simulink model "buenoensam"  (R2013a)
settings: Solver=ode5  StartTime=0.0  StopTime=40  FixedStep=.01  RelTol=1e-3
values from neighbouring files (symbols this model uses):
  g = 9.81    [miosinlazoalgebraico1.m]    (also in proyectoy6.m)
  theta2 = (m2*lc2*lc2)+I2    (= 0.00775807)    [miosinlazoalgebraico1.m]    (also in proyectoy6.m = 0.00125168)
  theta3 = (m2*l1*lc2)    (= 0.008897)    [miosinlazoalgebraico1.m]    (also in proyectoy6.m = 0.00091872)
  theta4 = (m1*lc1)+(m2*l1)    (= 0.495148)    [miosinlazoalgebraico1.m]    (also in proyectoy6.m = 0.014993)
  theta5 = (m2*lc2)    (= 0.044485)    [miosinlazoalgebraico1.m]    (also in proyectoy6.m = 0.008352)
undefined symbols (not defined in the file or in its folder): base, buenoensam, Pieza2, Pieza3, RootGround, RootPart, theta1
libraries: mblibv1 x14, fuzblock x4
settings Model: Creator=Daniel  LastModifiedBy=Daniel
settings SolverCC: MaxConsecutiveZCs=100000
settings SimMechanicsCC: VisOnUpdateDiagram=on  VisDuringSimulation=on

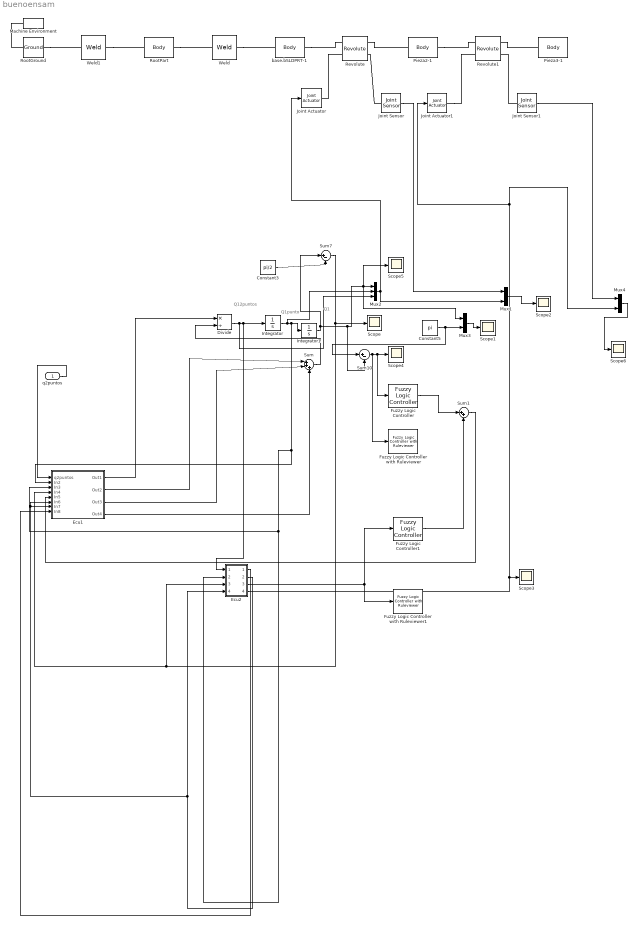
== system buenoensam ==
  note: Q1
  note: Q1punto
  note: Q12puntos
  q2puntos : Inport
  Constant3 : Constant  Value=pi/2
  Constant5 : Constant  Value=pi
  Divide : Product  Inputs=*/
  Ecu1 : Subsystem
  Ecu2 : Subsystem
  Fuzzy Logic Controller : fuzblock/Fuzzy Logic  Controller  fis=wero2P1
  Fuzzy Logic Controller with Ruleviewer : fuzblock/Fuzzy Logic  Controller  with Ruleviewer  fismatrix=wero2P1  Ts=2
  Fuzzy Logic Controller with Ruleviewer1 : fuzblock/Fuzzy Logic  Controller  with Ruleviewer  fismatrix=wero2P2  Ts=2
  Fuzzy Logic Controller1 : fuzblock/Fuzzy Logic  Controller  fis=wero2P2
  Integrator : Integrator
  Integrator1 : Integrator
  Joint Actuator : mblibv1/Sensors &  Actuators/Joint Actuator  UpdateFromCAD=off  PhysicalDomain=Mechanical  PortType=blob  ActuationStyle=Motion  AngleUnits=rad  ArcVelocityUnits=rad/s  ArcAccelerationUnits=rad/s^2  CoordPositionUnits=m  VelocityUnits=m/s  AccelerationUnits=m/s^2  ForceUnits=N  TorqueUnits=N*m  ActiveIO=on  Width=3  DialogClass=MechanicalActuatorBlock  Primitive=R1  ReferenceFrame=Absolute (World)
  Joint Actuator1 : mblibv1/Sensors &  Actuators/Joint Actuator  UpdateFromCAD=off  PhysicalDomain=Mechanical  PortType=blob  ActuationStyle=Motion  AngleUnits=rad  ArcVelocityUnits=rpm  ArcAccelerationUnits=rad/s^2  CoordPositionUnits=m  VelocityUnits=m/s  AccelerationUnits=m/s^2  ForceUnits=N  TorqueUnits=N*m  ActiveIO=on  Width=3  DialogClass=MechanicalActuatorBlock  Primitive=R1  ReferenceFrame=Absolute (World)
  Joint Sensor : mblibv1/Sensors &  Actuators/Joint Sensor  UpdateFromCAD=off  PhysicalDomain=Mechanical  PortType=blob  Muxed=on  Pose=off  Angle=on  AngleUnits=rad  ArcVelocity=off  ArcVelocityUnits=deg/s  ArcAcceleration=off  ArcAccelerationUnits=deg/s^2  CoordPosition=on  CoordPositionUnits=m  Velocity=off  VelocityUnits=m/s  Acceleration=off  AccelerationUnits=m/s^2  Quaternion=on  QuaternionDT=off  QuaternionDDT=off  QuaternionUnits=off  OutputVector=[1]  ActiveIO=on  Width=1  DialogClass=MechanicalSensorBlock  Primitive=R1  Force=off  ForceUnits=N  Torque=off  TorqueUnits=N*m  ReferenceFrame=Absolute (World)  ReactionSensedSide=Base  ReactionReferenceFrame=Absolute (World)  ReactionForce=off  ReactionForceUnits=N  ReactionMoment=off  ReactionMomentUnits=N*m
  Joint Sensor1 : mblibv1/Sensors &  Actuators/Joint Sensor  UpdateFromCAD=off  PhysicalDomain=Mechanical  PortType=blob  Muxed=on  Pose=off  Angle=on  AngleUnits=deg  ArcVelocity=off  ArcVelocityUnits=deg/s  ArcAcceleration=off  ArcAccelerationUnits=deg/s^2  CoordPosition=on  CoordPositionUnits=m  Velocity=off  VelocityUnits=m/s  Acceleration=off  AccelerationUnits=m/s^2  Quaternion=on  QuaternionDT=off  QuaternionDDT=off  QuaternionUnits=off  OutputVector=[1]  ActiveIO=on  Width=1  DialogClass=MechanicalSensorBlock  Primitive=R1  Force=off  ForceUnits=N  Torque=off  TorqueUnits=N-m  ReferenceFrame=Absolute (World)  ReactionSensedSide=Base  ReactionReferenceFrame=Absolute (World)  ReactionForce=off  ReactionForceUnits=N  ReactionMoment=off  ReactionMomentUnits=N-m
  Machine Environment : mblibv1/Bodies/Machine Environment  PortType=env  PhysicalDomain=Mechanical  DialogTemplateClass=MECH.MachineEnvironment  SyncWhenCopied=off  Gravity=[0 -9.81 0]  GravityUnits=m/s^2  GravityAsSignal=off  Dimensionality=Auto-detect  AnalysisType=Forward dynamics  LinearAssemblyTolerance=1e-3  LinearAssemblyToleranceUnits=m  AngularAssemblyTolerance=1e-3  AngularAssemblyToleranceUnits=rad  ConstraintSolverType=Stabilizing  ConstraintRelTolerance=1e-4  ConstraintAbsTolerance=1e-4  UseRobustSingularityHandling=off  RedundancyAnalysisToleranceType=Automatically select tolerance  RedundancyAnalysisTolerance=1e-14  StatePerturbationType=Fixed  PerturbationSize=1e-5  VisualizeMachine=on  BodyVisualizationType=Use model default body geometries  BodyColorSelMode=Use model default  DefaultBodyColor=[1 0 0]
  Mux1 : Mux  Inputs=2
  Mux2 : Mux  Inputs=3
  Mux3 : Mux  Inputs=2
  Mux4 : Mux  Inputs=2
  Pieza2-1 : mblibv1/Bodies/Body  LConnTagsString=CS2  RConnTagsString=CS3  UpdateFromCAD=on  PMImportedID=Pieza2-1  DialogClass=MechanicalBodyBlock  Mass=0.734204  MassUnits=kg  InertiaUnits=kg*m^2  Inertia=[0.000264247,2.83059e-10,-6.28102e-08;2.83059e-10,0.0127231,5.8833e-11;-6.28102e-08,5.8833e-11,0.0126365]  Shape=Cylinder  ShapeDims=[1 1]  ShapeUnits=m  ShapeUse=false  Density=1  DensityUnits=kg/m^3  DensityUse=false  GraphicsMode=GFXFILE  GraphicsFileName=buenoensam - Pieza2-1.STL  BodyColorSelMode=COLORPALETTE  BodyColor=[1;1;0]  AttachedToCS=CS1  CG=Right$CG$[-0.0307943 -0.183465 0.38735]$WORLD$WORLD$m$[0.0349053 0 -0.999391;-0.999391 0 -0.0349053;0 1 0]$3x3 Transform$rad$WORLD$false$Pieza2-1::CG(AUTOGEN)  WorkingFrames=Right$CS1$[-0.0615922 -0.0278733 0.3683]$WORLD$WORLD$m$[0.0349053 0 -0.999391;-0.999391 0 -0.0349053;0 1 0]$3x3 Transform$rad$WORLD$false$Pieza2-1::CS1(AUTOGEN)#Left$CS2$[-0.0384461 0.0361919 0.3683]$WORLD$WORLD$m$[1 0 0;0 1 0;0 0 1]$3x3 Transform$rad$WORLD$true$Pieza2-1:-:base.bSLDPRT-1::Pieza2-1(AUTOGEN)#Right$CS3$[-0.0234804 -0.394088 0.3683]$WORLD$WORLD$m$[1 0 0;0 1 0;0 0 1]$3x3 Transform$rad$WORLD$true$Pieza2-1:-:Pieza3-1::Pieza2-1(AUTOGEN)  CGPos=[-0.0307943 -0.183465 0.38735]  CGRot=[0.0349053 0 -0.999391;-0.999391 0 -0.0349053;0 1 0]  CS0Pos=[]  CS0Rot=[]  CS1Pos=[-0.0615922 -0.0278733 0.3683]  CS1Rot=[0.0349053 0 -0.999391;-0.999391 0 -0.0349053;0 1 0]  CS2Pos=[-0.0384461 0.0361919 0.3683]  CS2Rot=[1 0 0;0 1 0;0 0 1]  CS3Pos=[-0.0234804 -0.394088 0.3683]  CS3Rot=[1 0 0;0 1 0;0 0 1]  CS4Pos=[]  CS4Rot=[]  CS5Pos=[]  CS5Rot=[]  CS6Pos=[]  CS6Rot=[]  CS7Pos=[]  CS7Rot=[]  CS8Pos=[]  CS8Rot=[]  CS9Pos=[]  CS9Rot=[]  CS10Pos=[]  CS10Rot=[]  CS11Pos=[]  CS11Rot=[]  CS12Pos=[]  CS12Rot=[]  CS13Pos=[]  CS13Rot=[]  CS14Pos=[]  CS14Rot=[]  CS15Pos=[]  CS15Rot=[]  CS16Pos=[]  CS16Rot=[]  CS17Pos=[]  CS17Rot=[]  CS18Pos=[]  CS18Rot=[]  CS19Pos=[]  CS19Rot=[]  CS20Pos=[]  CS20Rot=[]
  Pieza3-1 : mblibv1/Bodies/Body  LConnTagsString=CS2  UpdateFromCAD=on  PMImportedID=Pieza3-1  DialogClass=MechanicalBodyBlock  Mass=0.784305  MassUnits=kg  InertiaUnits=kg*m^2  Inertia=[0.000374519,0.000457935,-7.77784e-07;0.000457935,0.0141418,4.97542e-08;-7.77784e-07,4.97542e-08,0.0141799]  Shape=Cylinder  ShapeDims=[1 1]  ShapeUnits=m  ShapeUse=false  Density=1  DensityUnits=kg/m^3  DensityUse=false  GraphicsMode=GFXFILE  GraphicsFileName=buenoensam - Pieza3-1.STL  BodyColorSelMode=COLORPALETTE  BodyColor=[0;1;1]  AttachedToCS=CS1  CG=Right$CG$[-0.0137132 -0.5717 0.352532]$WORLD$WORLD$m$[0.0550174 0 -0.998485;-0.998485 0 -0.0550174;0 1 0]$3x3 Transform$rad$WORLD$false$Pieza3-1::CG(AUTOGEN)  WorkingFrames=Right$CS1$[-0.0453321 -0.458607 0.3302]$WORLD$WORLD$m$[0.0550174 0 -0.998485;-0.998485 0 -0.0550174;0 1 0]$3x3 Transform$rad$WORLD$false$Pieza3-1::CS1(AUTOGEN)#Left$CS2$[-0.0234804 -0.394088 0.3683]$WORLD$WORLD$m$[1 0 0;0 1 0;0 0 1]$3x3 Transform$rad$WORLD$true$Pieza2-1:-:Pieza3-1::Pieza3-1(AUTOGEN)  CGPos=[-0.0137132 -0.5717 0.352532]  CGRot=[0.0550174 0 -0.998485;-0.998485 0 -0.0550174;0 1 0]  CS0Pos=[]  CS0Rot=[]  CS1Pos=[-0.0453321 -0.458607 0.3302]  CS1Rot=[0.0550174 0 -0.998485;-0.998485 0 -0.0550174;0 1 0]  CS2Pos=[-0.0234804 -0.394088 0.3683]  CS2Rot=[1 0 0;0 1 0;0 0 1]  CS3Pos=[]  CS3Rot=[]  CS4Pos=[]  CS4Rot=[]  CS5Pos=[]  CS5Rot=[]  CS6Pos=[]  CS6Rot=[]  CS7Pos=[]  CS7Rot=[]  CS8Pos=[]  CS8Rot=[]  CS9Pos=[]  CS9Rot=[]  CS10Pos=[]  CS10Rot=[]  CS11Pos=[]  CS11Rot=[]  CS12Pos=[]  CS12Rot=[]  CS13Pos=[]  CS13Rot=[]  CS14Pos=[]  CS14Rot=[]  CS15Pos=[]  CS15Rot=[]  CS16Pos=[]  CS16Rot=[]  CS17Pos=[]  CS17Rot=[]  CS18Pos=[]  CS18Rot=[]  CS19Pos=[]  CS19Rot=[]  CS20Pos=[]  CS20Rot=[]
  Revolute : mblibv1/Joints/Revolute  LConnTagsString=__newl0|SA1  RConnTagsString=__newr0|SA1  UpdateFromCAD=on  PMImportedID=Pieza2-1:-:base.bSLDPRT-1  NumSAPorts=2  CutJoint=off  MarkAsCut=off  Primitives=prismatic  PrimitiveProps=R1$World$[0,0,-1]$revolute  DialogClass=JointBlock  R1Axis=[0,0,-1]
  Revolute1 : mblibv1/Joints/Revolute  LConnTagsString=__newl0|SA1  RConnTagsString=__newr0|SA1  UpdateFromCAD=on  PMImportedID=Pieza2-1:-:Pieza3-1  NumSAPorts=2  CutJoint=off  MarkAsCut=off  Primitives=prismatic  PrimitiveProps=R1$World$[0,0,1]$revolute  DialogClass=JointBlock  R1Axis=[0,0,1]
  RootGround : mblibv1/Bodies/Ground  UpdateFromCAD=on  PMImportedID=RootGround  LeftPortType=env  RightPortType=workingframe  PhysicalDomain=Mechanical  DialogClass=GroundBlock  CoordPosition=[-0.0313325,-0.14828,0.31783]  CoordPositionUnits=m  StateVectorMgrId=0  MachineId=[1 0]  ShowEnvPort=on
  RootPart : mblibv1/Bodies/Body  LConnTagsString=CS3  RConnTagsString=CS2  UpdateFromCAD=on  PMImportedID=buenoensam/RootPart  DialogClass=MechanicalBodyBlock  Mass=0  MassUnits=kg  InertiaUnits=kg*m^2  Inertia=[0,0,0;0,0,0;0,0,0]  Shape=Cylinder  ShapeDims=[1 1]  ShapeUnits=m  ShapeUse=false  Density=1  DensityUnits=kg/m^3  DensityUse=false  GraphicsMode=MACHINE_DEFAULT  BodyColorSelMode=MACHINE_DEFAULT  BodyColor=[1;0;0]  AttachedToCS=CS1  CG=Right$CG$[-0.0313325 -0.14828 0.31783]$WORLD$WORLD$m$[1 0 0;0 1 0;0 0 1]$3x3 Transform$rad$WORLD$false$buenoensam/RootPart::CG(AUTOGEN)  WorkingFrames=Right$CS1$[0 0 0]$WORLD$WORLD$m$[1 0 0;0 1 0;0 0 1]$3x3 Transform$rad$WORLD$false$buenoensam/RootPart::CS1(AUTOGEN)#Right$CS2$[-0.0384461 0.0308496 0.278664]$WORLD$WORLD$m$[1 0 0;0 1 0;0 0 1]$3x3 Transform$rad$WORLD$true$base.bSLDPRT-1:-:buenoensam/RootPart::buenoensam/RootPart(AUTOGEN)#Left$CS3$[-0.0313325 -0.14828 0.31783]$WORLD$WORLD$m$[1 0 0;0 1 0;0 0 1]$3x3 Transform$rad$WORLD$true$RootGround:-:buenoensam/RootPart::buenoensam/RootPart(AUTOGEN)  CGPos=[-0.0313325 -0.14828 0.31783]  CGRot=[1 0 0;0 1 0;0 0 1]  CS0Pos=[]  CS0Rot=[]  CS1Pos=[0 0 0]  CS1Rot=[1 0 0;0 1 0;0 0 1]  CS2Pos=[-0.0384461 0.0308496 0.278664]  CS2Rot=[1 0 0;0 1 0;0 0 1]  CS3Pos=[-0.0313325 -0.14828 0.31783]  CS3Rot=[1 0 0;0 1 0;0 0 1]  CS4Pos=[]  CS4Rot=[]  CS5Pos=[]  CS5Rot=[]  CS6Pos=[]  CS6Rot=[]  CS7Pos=[]  CS7Rot=[]  CS8Pos=[]  CS8Rot=[]  CS9Pos=[]  CS9Rot=[]  CS10Pos=[]  CS10Rot=[]  CS11Pos=[]  CS11Rot=[]  CS12Pos=[]  CS12Rot=[]  CS13Pos=[]  CS13Rot=[]  CS14Pos=[]  CS14Rot=[]  CS15Pos=[]  CS15Rot=[]  CS16Pos=[]  CS16Rot=[]  CS17Pos=[]  CS17Rot=[]  CS18Pos=[]  CS18Rot=[]  CS19Pos=[]  CS19Rot=[]  CS20Pos=[]  CS20Rot=[]
  Scope{,1..6} (7 alike) : Scope
      Scope settings: TimeRange=15  YMin=1.5707963267948  YMax=1.5707963267956
      Scope1 settings: TimeRange=15  YMin=1.5707963267948  YMax=1.5707963267956  SaveName=ScopeData5
      Scope2 settings: YMin=-1.2e+17  YMax=7e+16  SaveName=ScopeData2
      Scope3 settings: YMin=-0.7  YMax=0.1  SaveName=ScopeData3
      Scope4 settings: YMin=398.84  YMax=399.05  SaveName=ScopeData4
      Scope5 settings: TimeRange=40  YMin=-596.787  YMax=-596.73  SaveName=ScopeData6
      Scope6 settings: YMin=-1.2e+17  YMax=7e+16  SaveName=ScopeData7
  Sum : Sum  Inputs=|+++
  Sum1 : Sum  Inputs=|++
  Sum10 : Sum  Inputs=|+-
  Sum7 : Sum  Inputs=|+-
  Weld : mblibv1/Joints/Weld  LConnTagsString=__newl0  RConnTagsString=__newr0  UpdateFromCAD=on  PMImportedID=base.bSLDPRT-1:-:buenoensam/RootPart  NumSAPorts=0  CutJoint=off  MarkAsCut=off  Primitives=weld  PrimitiveProps=W$WORLD$[0.57735,0.57735,0.57735]$weld  DialogClass=JointBlock  WAxis=[0.57735,0.57735,0.57735]
  Weld1 : mblibv1/Joints/Weld  LConnTagsString=__newl0  RConnTagsString=__newr0  UpdateFromCAD=on  PMImportedID=RootGround:-:buenoensam/RootPart  NumSAPorts=0  CutJoint=off  MarkAsCut=off  Primitives=weld  PrimitiveProps=W$WORLD$[0.57735,0.57735,0.57735]$weld  DialogClass=JointBlock  WAxis=[0.57735,0.57735,0.57735]
  base.bSLDPRT-1 : mblibv1/Bodies/Body  LConnTagsString=CS2  RConnTagsString=CS3  UpdateFromCAD=on  PMImportedID=base.bSLDPRT-1  DialogClass=MechanicalBodyBlock  Mass=1.99812  MassUnits=kg  InertiaUnits=kg*m^2  Inertia=[0.0110019,0,0;0,0.0129359,-0.000127709;0,-0.000127709,0.00347297]  Shape=Cylinder  ShapeDims=[1 1]  ShapeUnits=m  ShapeUse=false  Density=1  DensityUnits=kg/m^3  DensityUse=false  GraphicsMode=GFXFILE  GraphicsFileName=buenoensam - base.bSLDPRT-1.STL  BodyColorSelMode=COLORPALETTE  BodyColor=[0;0;1]  AttachedToCS=CS1  CG=Right$CG$[-0.0384461 0.0308496 0.278664]$WORLD$WORLD$m$[1 0 0;0 1 0;0 0 1]$3x3 Transform$rad$WORLD$false$base.bSLDPRT-1::CG(AUTOGEN)  WorkingFrames=Right$CS1$[-0.0384461 -0.00190807 0.1651]$WORLD$WORLD$m$[1 0 0;0 1 0;0 0 1]$3x3 Transform$rad$WORLD$false$base.bSLDPRT-1::CS1(AUTOGEN)#Left$CS2$[-0.0384461 0.0308496 0.278664]$WORLD$WORLD$m$[1 0 0;0 1 0;0 0 1]$3x3 Transform$rad$WORLD$true$base.bSLDPRT-1:-:buenoensam/RootPart::base.bSLDPRT-1(AUTOGEN)#Right$CS3$[-0.0384461 0.0361919 0.3683]$WORLD$WORLD$m$[1 0 0;0 1 0;0 0 1]$3x3 Transform$rad$WORLD$true$Pieza2-1:-:base.bSLDPRT-1::base.bSLDPRT-1(AUTOGEN)  CGPos=[-0.0384461 0.0308496 0.278664]  CGRot=[1 0 0;0 1 0;0 0 1]  CS0Pos=[]  CS0Rot=[]  CS1Pos=[-0.0384461 -0.00190807 0.1651]  CS1Rot=[1 0 0;0 1 0;0 0 1]  CS2Pos=[-0.0384461 0.0308496 0.278664]  CS2Rot=[1 0 0;0 1 0;0 0 1]  CS3Pos=[-0.0384461 0.0361919 0.3683]  CS3Rot=[1 0 0;0 1 0;0 0 1]  CS4Pos=[]  CS4Rot=[]  CS5Pos=[]  CS5Rot=[]  CS6Pos=[]  CS6Rot=[]  CS7Pos=[]  CS7Rot=[]  CS8Pos=[]  CS8Rot=[]  CS9Pos=[]  CS9Rot=[]  CS10Pos=[]  CS10Rot=[]  CS11Pos=[]  CS11Rot=[]  CS12Pos=[]  CS12Rot=[]  CS13Pos=[]  CS13Rot=[]  CS14Pos=[]  CS14Rot=[]  CS15Pos=[]  CS15Rot=[]  CS16Pos=[]  CS16Rot=[]  CS17Pos=[]  CS17Rot=[]  CS18Pos=[]  CS18Rot=[]  CS19Pos=[]  CS19Rot=[]  CS20Pos=[]  CS20Rot=[]
  wires:
  Divide/1 -> Mux2/3, Ecu2/1(In1), Integrator/1
  Integrator/1 -> Mux2/2, Integrator1/1, Ecu1/2(In2), Ecu1/3(In3), Ecu2/2(In2)
  Sum/1 -> Divide/2
  Mux2/1 -> Joint Actuator/1, Mux1/2
  Joint Sensor/1 -> Mux1/1
  Mux1/1 -> Scope2/1
  Joint Sensor1/1 -> Mux4/1
  Constant3/1 -> Sum7/2
  Integrator1/1 -> Sum10/2, Scope5/1, Mux3/1, Mux2/1, Sum7/1
  Sum7/1 -> Ecu1/4(In4), Ecu2/3(In3), Scope/1
  Constant5/1 -> Sum10/1, Mux3/2
  Sum10/1 -> Fuzzy Logic Controller with Ruleviewer/1, Fuzzy Logic Controller/1, Scope4/1
  Ecu2/2(Out2) -> Ecu1/6(In6), Ecu1/7(In7), Ecu2/4(In4)
  Ecu2/4(Out4) -> Joint Actuator1/1, Mux4/2, Scope3/1
  q2puntos/1 -> Ecu1/1(q2puntos)
  Ecu2/1(Out1) -> Ecu1/8(In8)
  Ecu1/1(Out1) -> Divide/1
  Ecu1/2(Out2) -> Sum/1
  Ecu1/3(Out3) -> Sum/2
  Ecu1/4(Out4) -> Sum/3
  Ecu2/3(Out3) -> Fuzzy Logic Controller with Ruleviewer1/1, Fuzzy Logic Controller1/1
  Fuzzy Logic Controller/1 -> Sum1/1
  Fuzzy Logic Controller1/1 -> Sum1/2
  Sum1/1 -> Ecu1/5(In5)
  Mux3/1 -> Scope1/1
  Mux4/1 -> Scope6/1
  connections:
  RootPart/RConn1 -- Weld/LConn1
  Weld/RConn1 -- base.bSLDPRT-1/LConn1
  base.bSLDPRT-1/RConn1 -- Revolute/LConn1
  Revolute/RConn1 -- Pieza2-1/LConn1
  Pieza2-1/RConn1 -- Revolute1/LConn1
  Revolute1/RConn1 -- Pieza3-1/LConn1
  RootGround/RConn1 -- Weld1/LConn1
  Weld1/RConn1 -- RootPart/LConn1
  RootGround/LConn1 -- Machine Environment/RConn1
  Joint Actuator/RConn1 -- Revolute/LConn2
  Joint Sensor/LConn1 -- Revolute/RConn2
  Joint Actuator1/RConn1 -- Revolute1/LConn2
  Joint Sensor1/LConn1 -- Revolute1/RConn2

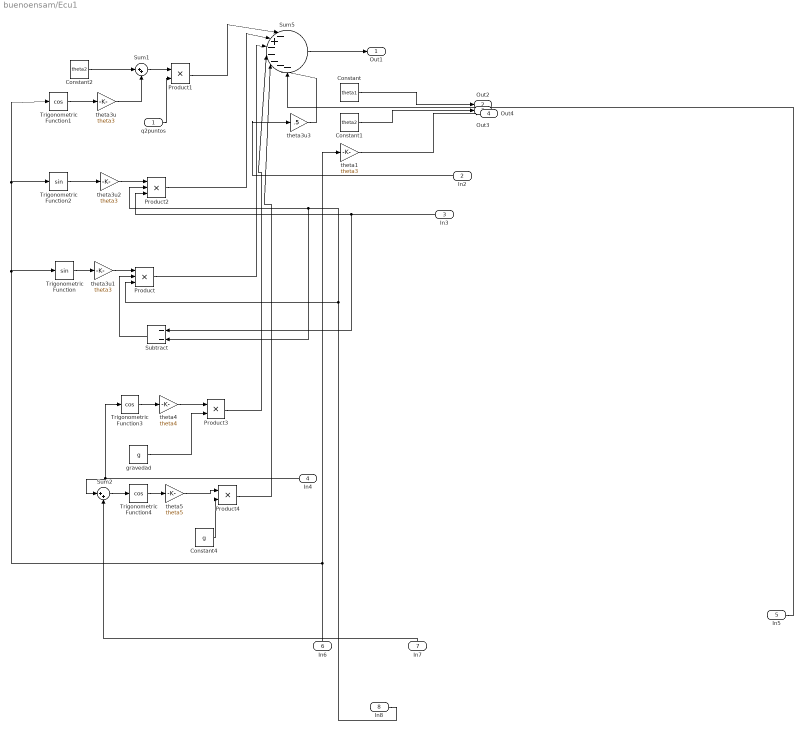
== system buenoensam/Ecu1 ==
  q2puntos : Inport
  In2 : Inport  Port=2
  In3 : Inport  Port=3
  In4 : Inport  Port=4
  In5 : Inport  Port=5
  In6 : Inport  Port=6
  In7 : Inport  Port=7
  In8 : Inport  Port=8
  Constant : Constant  Value=theta1
  Constant1 : Constant  Value=theta2
  Constant2 : Constant  Value=theta2
  Constant4 : Constant  Value=g
  Product : Product  Inputs=3
  Product1 : Product
  Product2 : Product  Inputs=3
  Product3 : Product
  Product4 : Product
  Subtract : Sum  Inputs=--
  Sum1 : Sum  Inputs=|++
  Sum2 : Sum  Inputs=|++
  Sum5 : Sum  Inputs=|-+-----
  Trigonometric Function : Trigonometry
  Trigonometric Function1 : Trigonometry  Operator=cos
  Trigonometric Function2 : Trigonometry
  Trigonometric Function3 : Trigonometry  Operator=cos
  Trigonometric Function4 : Trigonometry  Operator=cos
  gravedad : Constant  Value=g
  theta1 : Gain  Gain=theta3
  theta3u : Gain  Gain=theta3
  theta3u1 : Gain  Gain=theta3
  theta3u2 : Gain  Gain=theta3
  theta3u3 : Gain  Gain=.5
  theta4 : Gain  Gain=theta4
  theta5 : Gain  Gain=theta5
  Out1 : Outport
  Out2 : Outport  Port=2
  Out3 : Outport  Port=3
  Out4 : Outport  Port=4
  wires:
  Constant2/1 -> Sum1/1
  theta3u/1 -> Sum1/2
  Trigonometric Function1/1 -> theta3u/1
  Sum1/1 -> Product1/1
  q2puntos/1 -> Product1/2
  Product1/1 -> Sum5/1
  Trigonometric Function2/1 -> theta3u2/1
  theta3u2/1 -> Product2/1
  Product2/1 -> Sum5/2
  Product/1 -> Sum5/3
  Trigonometric Function/1 -> theta3u1/1
  theta3u1/1 -> Product/1
  Product3/1 -> Sum5/4
  Trigonometric Function3/1 -> theta4/1
  theta4/1 -> Product3/1
  gravedad/1 -> Product3/2
  Product4/1 -> Sum5/5
  Trigonometric Function4/1 -> theta5/1
  Sum2/1 -> Trigonometric Function4/1
  theta5/1 -> Product4/1
  Constant4/1 -> Product4/2
  Constant/1 -> Out2/1
  Constant1/1 -> Out3/1
  theta1/1 -> Out4/1
  Sum5/1 -> Out1/1
  Subtract/1 -> Product/2
  theta3u3/1 -> Sum5/6
  In5/1 -> Sum5/7
  In3/1 -> Subtract/1, Product2/3
  In4/1 -> Trigonometric Function3/1, Sum2/1
  In7/1 -> Sum2/2
  In2/1 -> theta3u3/1
  In6/1 -> theta1/1, Trigonometric Function/1, Trigonometric Function2/1, Trigonometric Function1/1
  In8/1 -> Subtract/2, Product2/2, Product/3

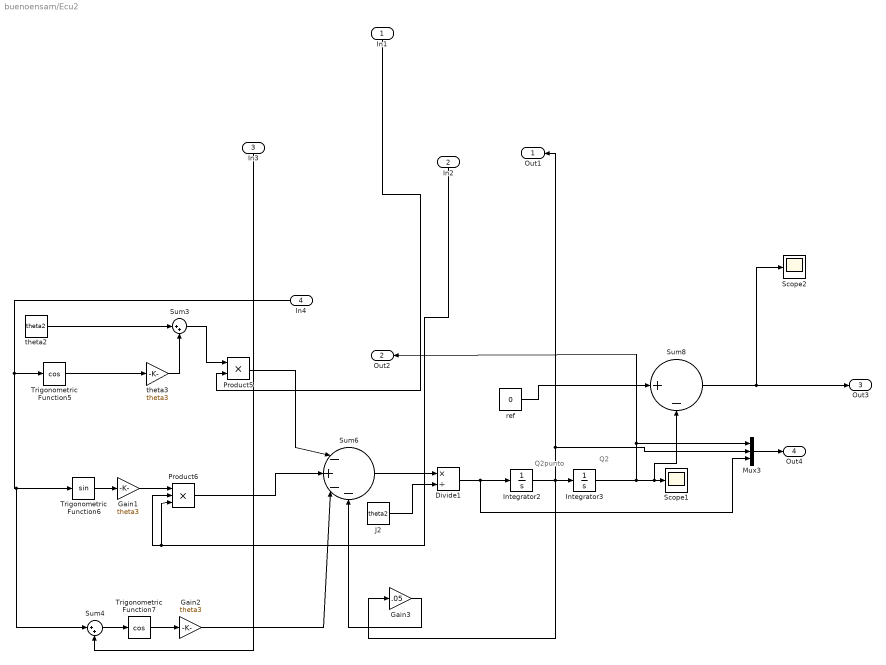
== system buenoensam/Ecu2 ==
  note: Q2
  note: Q2punto
  In1 : Inport
  In2 : Inport  Port=2
  In3 : Inport  Port=3
  In4 : Inport  Port=4
  Divide1 : Product  Inputs=*/
  Gain1 : Gain  Gain=theta3
  Gain2 : Gain  Gain=theta3
  Gain3 : Gain  Gain=.05
  Integrator2 : Integrator
  Integrator3 : Integrator
  J2 : Constant  Value=theta2
  Mux3 : Mux  Inputs=3
  Product5 : Product
  Product6 : Product  Inputs=3
  Scope1 : Scope
      settings: YMin=1.8293  YMax=1.8313
  Scope2 : Scope
      settings: YMin=-1.8417  YMax=-1.8403  SaveName=ScopeData9
  Sum3 : Sum  Inputs=|++
  Sum4 : Sum  Inputs=|++
  Sum6 : Sum  Inputs=|-+--
  Sum8 : Sum  Inputs=|+-
  Trigonometric Function5 : Trigonometry  Operator=cos
  Trigonometric Function6 : Trigonometry
  Trigonometric Function7 : Trigonometry  Operator=cos
  ref : Constant  Value=0
  theta2 : Constant  Value=theta2
  theta3 : Gain  Gain=theta3
  Out1 : Outport
  Out2 : Outport  Port=2
  Out3 : Outport  Port=3
  Out4 : Outport  Port=4
  wires:
  Trigonometric Function5/1 -> theta3/1
  theta2/1 -> Sum3/1
  theta3/1 -> Sum3/2
  Sum3/1 -> Product5/1
  Product5/1 -> Sum6/1
  Trigonometric Function6/1 -> Gain1/1
  Product6/1 -> Sum6/2
  Gain1/1 -> Product6/1
  Gain2/1 -> Sum6/3
  Trigonometric Function7/1 -> Gain2/1
  Sum4/1 -> Trigonometric Function7/1
  Sum6/1 -> Divide1/1
  Divide1/1 -> Mux3/3, Integrator2/1
  J2/1 -> Divide1/2
  Gain3/1 -> Sum6/4
  Integrator2/1 -> Gain3/1, Out1/1, Mux3/2, Integrator3/1
  Mux3/1 -> Out4/1
  ref/1 -> Sum8/1
  Integrator3/1 -> Out2/1, Mux3/1, Sum8/2, Scope1/1
  Sum8/1 -> Scope2/1, Out3/1
  In4/1 -> Sum4/1, Trigonometric Function6/1, Trigonometric Function5/1
  In3/1 -> Sum4/2
  In2/1 -> Product6/3, Product6/2
  In1/1 -> Product5/2
